simulink model "nsdynamic_Energy"  (R2021b)
settings: Solver=ode4  StartTime=0.0  StopTime=10.0  RelTol=1e-3
InitFcn:
  | initialization
undefined symbols (not defined in the file or in its folder): dynNS_Energy, trajectory
settings Model: Creator=AzamaoZ  LastModifiedBy=AzamaoZ

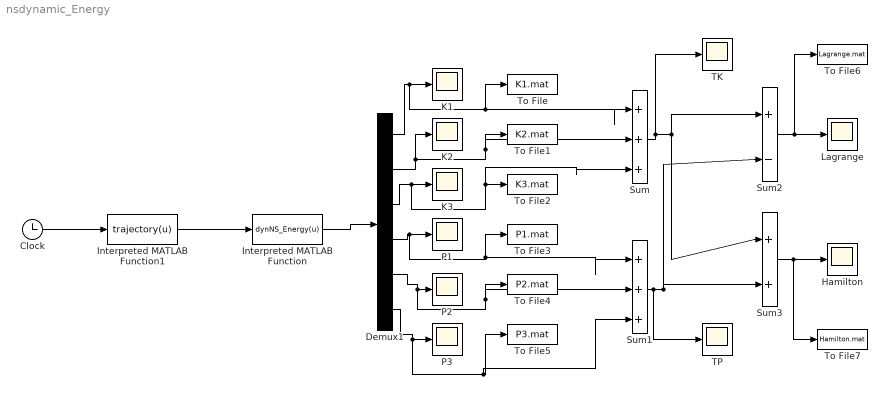
== system nsdynamic_Energy ==
  Clock : Clock
  Demux1 : Demux  Outputs=6
  Hamilton : Scope
  Interpreted MATLAB Function : MATLABFcn  MATLABFcn=dynNS_Energy(u)  OutputDimensions=6
  Interpreted MATLAB Function1 : MATLABFcn  MATLABFcn=trajectory(u)
  K1 : Scope
  K2 : Scope
  K3 : Scope
  Lagrange : Scope
  P1 : Scope
  P2 : Scope
  P3 : Scope
  Sum : Sum  Inputs=|+++
  Sum1 : Sum  Inputs=|+++
  Sum2 : Sum  Inputs=|+-
  Sum3 : Sum  Inputs=|++
  TK : Scope
  TP : Scope
  To File : ToFile  Filename=K1.mat  MatrixName=K1  SaveFormat=Timeseries
  To File1 : ToFile  Filename=K2.mat  MatrixName=K2  SaveFormat=Timeseries
  To File2 : ToFile  Filename=K3.mat  MatrixName=K3  SaveFormat=Timeseries
  To File3 : ToFile  Filename=P1.mat  MatrixName=P1  SaveFormat=Timeseries
  To File4 : ToFile  Filename=P2.mat  MatrixName=P2  SaveFormat=Timeseries
  To File5 : ToFile  Filename=P3.mat  MatrixName=P3  SaveFormat=Timeseries
  To File6 : ToFile  Filename=Lagrange.mat  MatrixName=Lagrange  SaveFormat=Timeseries
  To File7 : ToFile  Filename=Hamilton.mat  MatrixName=Hamilton  SaveFormat=Timeseries
  wires:
  Interpreted MATLAB Function/1 -> Demux1/1
  Clock/1 -> Interpreted MATLAB Function1/1
  Demux1/1 -> Sum/1, To File/1, K1/1
  Demux1/2 -> K2/1, Sum/2, To File1/1
  Demux1/4 -> Sum1/1, To File3/1, P1/1
  Demux1/6 -> Sum1/3, To File5/1, P3/1
  Demux1/5 -> Sum1/2, To File4/1, P2/1
  Demux1/3 -> Sum/3, To File2/1, K3/1
  Interpreted MATLAB Function1/1 -> Interpreted MATLAB Function/1
  Sum1/1 -> TP/1, Sum2/2, Sum3/2
  Sum/1 -> TK/1, Sum3/1, Sum2/1
  Sum2/1 -> To File6/1, Lagrange/1
  Sum3/1 -> To File7/1, Hamilton/1
